simulink model "fMPC"  (R2018b)
settings: Solver=FixedStepDiscrete  StartTime=0.0  StopTime=10  FixedStep=0.5  RelTol=1e-3
undefined symbols (not defined in the file): A, B, m, nm, R, T, x0
settings Model: DataDictionary=f_mpc.sldd  Creator=bradyplanden  LastModifiedBy=bradyplanden
settings SFSimCC: SimCustomHeaderCode="#include \"f_mpc.h\""  SimUserSources=src/f_mpc.c  SimUserIncludeDirs=/usr/lib  SimUserLibraries=libblas.dylib liblapack.dylib  SimAnalyzeCustomCode=on
settings RTWCC: RTWUseSimCustomCode=on  CustomHeaderCode="#include \"f_mpc.h\""  CustomInclude=/usr/lib  CustomSource=src/f_mpc.c  CustomLibrary=libblas.dylib liblapack.dylib

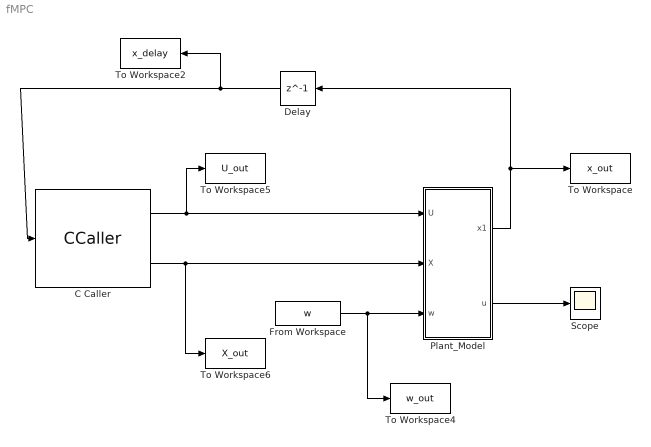
== system fMPC ==
  C Caller : CCaller  FunctionName=fmpcsolve  PortSpecificationStruct="%)30     .    ,\"    8    (     @         %    \"    !8    !     0         %  0 \"0    $    V    07)G3F%M90  4&]R=$YA;64 4V-O<&4     26YD97@     5'EP90      4VEZ90         .    ,     8    (    !          %    \"     $    !     0         0  $ 00    X    P    !@    @    $          4    (     0    $    !         !   0!!    #@   $     &    \"     0         !0    @    !    \"0    $         $     D   !0 ...(+10750 chars)"  A=A  B=B  At=At  Bt=Bt  eyen=eyen  eyem=eyem  Q=Q  R=R  Qf=Qf  zmax=zmax  zmin=zmin  z0=z0  T=T  n=n  m=m  nz=nz  niters=niters  kappa=kappa  z=z
  Delay : Delay  DelayLength=1  InitialCondition=x0  InputProcessing=Inherited
  From Workspace : FromWorkspace  VariableName=w  SampleTime=0.5  OutputAfterFinalValue=Setting to zero
  Plant_Model : MATLAB Function  TreatAsAtomicUnit=on
  Scope : Scope
  To Workspace : ToWorkspace  VariableName=x_out  SaveFormat=Structure With Time  SampleTime=-1
  To Workspace2 : ToWorkspace  VariableName=x_delay  SaveFormat=Structure With Time  SampleTime=-1
  To Workspace4 : ToWorkspace  VariableName=w_out  SaveFormat=Structure With Time  SampleTime=-1
  To Workspace5 : ToWorkspace  VariableName=U_out  SaveFormat=Structure With Time  SampleTime=-1
  To Workspace6 : ToWorkspace  VariableName=X_out  SaveFormat=Structure With Time  SampleTime=-1
  wires:
  C Caller/1 -> Plant_Model/1(U), To Workspace5/1
  C Caller/2 -> Plant_Model/2(X), To Workspace6/1
  Delay/1 -> C Caller/1, To Workspace2/1
  Plant_Model/1(x1) -> Delay/1, To Workspace/1
  From Workspace/1 -> To Workspace4/1, Plant_Model/3(w)
  Plant_Model/2(u) -> Scope/1

== matlab function fMPC/Plant_Model ==
  data: U input; X input; x1 output; A parameter; nm parameter; T parameter; B parameter; w input; u output
function [x1,u]  = Plant(U,X,A,nm, T, B, w)

%Taking the first entry of U
u = U(:,1);

%Taking the first entry of X
x = X(:,1);

%Updating State Equation
x1 =A*x+B*u+w;
